simulink model "sf_atomic_sensor_pair"  (Simulink 7.6)
settings: Solver=FixedStepDiscrete  StartTime=0.0  StopTime=Inf  FixedStep=1  RelTol=1e-3
libraries: simulink x2, sf_atomic_sensor_lib x2
settings Model: Creator=The MathWorks Inc.
settings SFSimCC: SimParseCustomCode=off

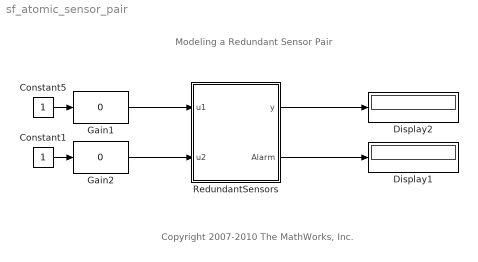
== system sf_atomic_sensor_pair ==
  note: Copyright 2007-2010 The MathWorks, Inc.
  note: Modeling a Redundant Sensor Pair
  Constant1 : Constant
  Constant5 : Constant
  Display1 : Display
  Display2 : Display
  Gain1 : simulink/Math Operations/Slider Gain  SystemSampleTime=-1  low=-200  gain=0  high=300
  Gain2 : simulink/Math Operations/Slider Gain  SystemSampleTime=-1  low=-200  gain=0  high=300
  RedundantSensors : Stateflow chart  TreatAsAtomicUnit=on
  wires:
  Constant5/1 -> Gain1/1
  Gain1/1 -> RedundantSensors/1(u1)
  Constant1/1 -> Gain2/1
  Gain2/1 -> RedundantSensors/2(u2)
  RedundantSensors/1(y) -> Display2/1
  RedundantSensors/2(Alarm) -> Display1/1

== stateflow chart RedundantSensors ==
  state Sensor1
  state Sensor2
  state Alarm
    en, du: y = 0;
  (default) -> Sensor1
  Sensor1 -> Sensor2 : [Sensor1.inFailed()]
  Sensor2 -> Alarm : [Sensor2.inFailed()]
  data: u1 input double; u2 input double; y output double; Alarm output boolean
